simulink library "psa_examples_lib"  (R2015a)
settings: Solver=ode45  StartTime=0.0  StopTime=10.0  RelTol=1e-3
libraries: libSimulators x1
settings Model: Creator=jcardena  LastModifiedBy=ecastill

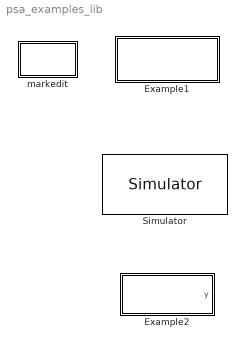
== system psa_examples_lib ==
  Example1 : Subsystem  mask{nwhts=0, wh_ts=600}
      mask prompts: nwhts "Numbers of the Units"; wh_ts "Sampling Time"
      settings: OpenFcn=read_simulated_unitIDs_example;
      mask Callback nwhts:
      | %keyboard;
      | nwh=get_param(gcb,'nwhts');
      | if nwh<1,
      |    nwh=1;
      |     set_param(gcb,'nwhts', 'nwh');
      | end;
  "Example2 " : Subsystem  mask{yVar='14B60'}
      mask prompts: yVar "Hexadecimal Output [evaluated]"
      mask init:
      | y = hex2dec(yVar);
      settings: DeleteFcn=slexUtilityCloseMaskExample(get_param(gcb, 'handle'));
  Simulator : libSimulators/Simulator  unitIDs=0  searchString='%20151209%'  db_name=HeatingUnits  db_username=sw_waterheaters  db_password=unb.sql.2015  msgError_edit=Connection successful
  markedit : Subsystem
      settings: OpenFcn=psa_examples_lib(get_param([gcs, '/Example2'], 'handle'),1);
      mask Display: disp('View\nMask')

== system psa_examples_lib/Example1 ==

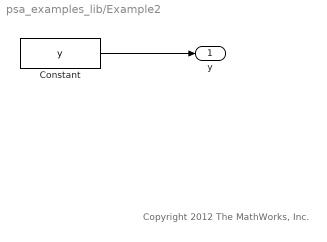
== system psa_examples_lib/Example2  ==
  note: Copyright 2012 The MathWorks, Inc.
  Constant : Constant  Value=y
  y : Outport
  wires:
  Constant/1 -> y/1

== system psa_examples_lib/markedit ==
